simulink model "CAT797_lateral_dynamics_open_loop_2024a"  (R2024a)
settings: Solver=ode4  StartTime=0.0  StopTime=10  FixedStep=0.001  RelTol=1e-3
PreLoadFcn:
  | addpath("G:\Control_Research\Autonomy_Mining_Dump_Truck\src\plant_model\lib")
libraries: lat_dyn_haul_00 x1
settings Model: DataDictionary=CAT_797F.sldd  Creator=marti343  LastModifiedBy=marti343
settings ConfigComp: CovBoundaryAbsTol=1.0e-5

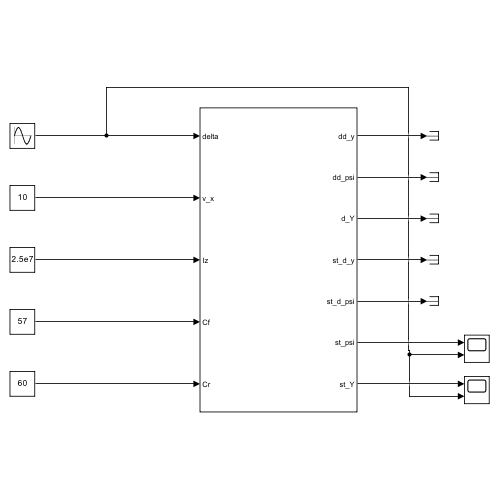
[thumbnail: Simulink's stored preview of the top-level diagram]
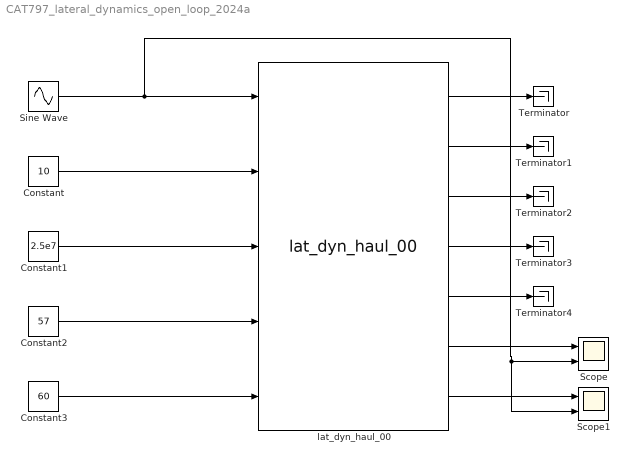
== system CAT797_lateral_dynamics_open_loop_2024a ==
  Constant : Constant  Value=10
  Constant1 : Constant  Value=2.5e7
  Constant2 : Constant  Value=57
  Constant3 : Constant  Value=60
  Scope : Scope  NumInputPorts=2
  Scope1 : Scope  NumInputPorts=2
  Sine Wave : Sin  Amplitude=20
  Terminator{,1..4} (5 alike) : Terminator
  lat_dyn_haul_00 : lat_dyn_haul_00/lat_dyn_haul_00  SystemSampleTime=-1  VariantActivationTime=update diagram  EmptyChoice=off  PassThrough=off  PassThroughVariantControl=(default)  EmptyChoiceVariantControl=(default)  AllowFlexibleInterface=on  Latency=0  AutoFrameSizeCalculation=off
  wires:
  Sine Wave/1 -> Scope1/2, Scope/2, lat_dyn_haul_00/1
  lat_dyn_haul_00/6 -> Scope/1
  lat_dyn_haul_00/7 -> Scope1/1
  lat_dyn_haul_00/1 -> Terminator/1
  lat_dyn_haul_00/2 -> Terminator1/1
  lat_dyn_haul_00/3 -> Terminator2/1
  lat_dyn_haul_00/4 -> Terminator3/1
  lat_dyn_haul_00/5 -> Terminator4/1
  Constant/1 -> lat_dyn_haul_00/2
  Constant1/1 -> lat_dyn_haul_00/3
  Constant2/1 -> lat_dyn_haul_00/4
  Constant3/1 -> lat_dyn_haul_00/5
